simulink model "Speed_Controller_Test_forTD"  (Simulink 6.6)
settings: Solver=ode4  SolverMode=SingleTasking  StartTime=0.0  StopTime=252  FixedStep=0.01  RelTol=1e-3
InitFcn:
  | tempomat_para
StopFcn:
  | clear;
values from neighbouring files (symbols this model uses):
  A = 1.9    [tempomat_para.m]
  a_Fzg_max = 2    [tempomat_para.m]
  a_Fzg_min = -2    [tempomat_para.m]
  cw = 0.32    [tempomat_para.m]
  gang = [1 2 3 4]    [tempomat_para.m]
  gang_vec = [1 2 3 4]    [tempomat_para.m]
  i_anteil = 5    [tempomat_para.m]
  i_d = 3.42    [tempomat_para.m]
  i_g = [3.91 2.17 1.37 1.00]    [tempomat_para.m]
  lambda_gang = [1.3 1.25  1.17  1.05]    [tempomat_para.m]
  m_Fzg = 1400    [tempomat_para.m]
  M_mot_max = [130 149 163 170 168 166 162 158 150 139 123 80]    [tempomat_para.m]
  M_mot_min = [0 -40]    [tempomat_para.m]
  n_mot0 = 1000    [tempomat_para.m]
  n_mot_max = 1000:500:6500    [tempomat_para.m]
  n_mot_min = [1000 6500]    [tempomat_para.m]
  p_anteil = 100    [tempomat_para.m]
  r_dyn = 0.28    [tempomat_para.m]
  rho = 1.202    [tempomat_para.m]
  t_sch = 0.2    [tempomat_para.m]
  TI = [block '/TI']    [PSTI_callback.m]
  v_Fzg_ms0 = 0    [tempomat_para.m]
undefined symbols (not defined in the file or in its folder): Drossel_mat, getdatatypespecs
libraries: simulink x116, fzgbib x3
(part 1 of 9)
settings Model: Creator=Abel  LastModifiedBy=Justyna
settings DataIOCC: LimitDataPoints=off  SignalLoggingName=sigsOut
settings OptimizationCC: BooleanDataType=off
settings DebuggingCC: SignalResolutionControl=TryResolveAllWithWarning  InheritedTsInSrcMsg=none  MultiTaskDSMMsg=warning  MultiTaskCondExecSysMsg=none  StrictBusMsg=None
settings RTWCC: IncludeERTFirstTime=on

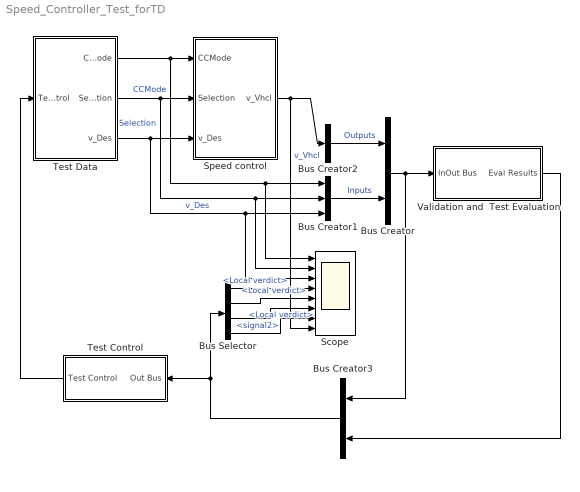
== system Speed_Controller_Test_forTD ==
  Bus Creator : BusCreator  Inputs=2
  Bus Creator1 : BusCreator  Inputs=3
  Bus Creator2 : BusCreator  Inputs=1
  Bus Creator3 : BusCreator  Orientation=left  Inputs=2
  Bus Selector : BusSelector  OutputSignals=signal2.signal1.signal1.signal1.signal1.Local verdict,signal2.signal1.signal1.signal1.signal2.Local verdict,signal2.signal1.signal2.signal1.signal1.Local verdict,signal2.signal2
  Scope : Scope  NumInputPorts=8
      settings: YMin=-5~-5~-5~-5~-5~-5~-5~-5  YMax=5~5~5~5~5~5~5~5  MaxDataPoints=5000000
  Speed control : Subsystem
  Test Control : Subsystem  Orientation=left
  Test Data : Subsystem
  Validation and  Test Evaluation : Subsystem  Description=Test evaluation system template. Create a new test evaluation system from this template.
  wires:
  Speed control/1(v_Vhcl) -> Bus Creator2/1, Scope/8  "v_Vhcl"
  Test Data/1(CCMode) -> Speed control/1(CCMode), Bus Creator1/1, Scope/1  "CCMode"
  Test Data/2(Selection) -> Speed control/2(Selection), Bus Creator1/2, Scope/2  "Selection"
  Bus Creator/1 -> Validation and  Test Evaluation/1(InOut Bus), Bus Creator3/1
  Bus Creator2/1 -> Bus Creator/1  "Outputs"
  Bus Creator1/1 -> Bus Creator/2  "Inputs"
  Test Data/3(v_Des) -> Speed control/3(v_Des), Scope/3, Bus Creator1/3  "v_Des"
  Bus Creator3/1 -> Test Control/1(Out Bus), Bus Selector/1
  Validation and  Test Evaluation/1(Eval Results) -> Bus Creator3/2
  Test Control/1(Test Control) -> Test Data/1(Test Control)
  Bus Selector/1 -> Scope/4  "<Local verdict>"
  Bus Selector/2 -> Scope/5  "<Local verdict>"
  Bus Selector/3 -> Scope/6  "<Local verdict>"
  Bus Selector/4 -> Scope/7  "<signal2>"

== system Speed_Controller_Test_forTD/Speed control ==
  CCMode : Inport
  Selection : Inport  Port=2
  v_Des : Inport  Port=3
  Bus Selector : BusSelector  OutputSignals=i_Total,n_Eng,a_Vhcl,v_Vhcl
  Compute SUC inputs : Subsystem  AncestorBlock=fzgbib/StellgroessenBerechnung BeschleunigungsBegrenzung
  Const : Constant
  Speed controller : Subsystem  AncestorBlock=fzgbib/GeschwindigkeitsRegelung
  Terminator1 : Terminator
  Terminator2 : Terminator
  Vehicle model : Subsystem
      mask Type: Vehicle Model
      mask Display: image(imread('car.jpg','jpg'),[0.05,0.2,0.9,0.6])
  "km/h -> m/s2" : Gain  Gain=1/3.6  SaturateOnIntegerOverflow=on
  "m/s2 -> km/h" : Gain  Gain=3.6  SaturateOnIntegerOverflow=on
  v_Vhcl : Outport
  wires:
  Speed controller/1(T) -> Compute SUC inputs/4(T)
  Vehicle model/1(FzgDaten) -> Bus Selector/1
  Bus Selector/1 -> Compute SUC inputs/1(i_Total)  "<i_Total>"
  Bus Selector/2 -> Compute SUC inputs/2(n_Eng)  "<n_Eng>"
  Bus Selector/3 -> Compute SUC inputs/3(a_Vhcl)  "<a_Vhcl>"
  Bus Selector/4 -> Speed controller/1(v_Vhcl), "m/s2 -> km/h"/1  "<v_Vhcl>"
  Vehicle model/2(M_Br_b) -> Terminator1/1
  Vehicle model/3(M_Mot_b) -> Terminator2/1
  Compute SUC inputs/1(SUC inputs) -> Vehicle model/1(StellgroessenTempomat), Vehicle model/3(StellgroessenFahrer)
  v_Des/1 -> "km/h -> m/s2"/1
  "m/s2 -> km/h"/1 -> v_Vhcl/1
  "km/h -> m/s2"/1 -> Speed controller/2(v_Des)
  Const/1 -> Vehicle model/2(TempomatFlag)
  Selection/1 -> Speed controller/3(Selection)
  CCMode/1 -> Speed controller/4(CCMode)

== system Speed_Controller_Test_forTD/Test Control ==
  Out Bus : Inport
  Bus Selector : BusSelector  OutputSignals=signal2.signal1.signal1.signal1.signal1.Local verdict
  Counter : Subsystem
  Memory : Memory
  OR : Logic  Operator=OR  Inputs=3  AllPortsSameDT=off  OutDataTypeMode=Boolean
  Switch : Switch  Criteria=u2 > Threshold
  error : simulink/Logic and Bit Operations/Compare To Constant  SystemSampleTime=-1  relop===  const=-1  LogicOutDataTypeMode=uint8  ZeroCross=off
  fail : simulink/Logic and Bit Operations/Compare To Constant  SystemSampleTime=-1  relop===  const=0  LogicOutDataTypeMode=uint8  ZeroCross=off
  pass : simulink/Logic and Bit Operations/Compare To Constant  SystemSampleTime=-1  relop===  const=1  LogicOutDataTypeMode=uint8  ZeroCross=off
  test case 1 : Constant
  test case 2 : Constant  Value=2
  Test Control : Outport
  wires:
  OR/1 -> Counter/1(In1), Counter/Trigger
  test case 1/1 -> Switch/3
  Out Bus/1 -> Bus Selector/1
  Switch/1 -> Test Control/1
  test case 2/1 -> Switch/1
  Counter/1(Out1) -> Switch/2
  Bus Selector/1 -> Memory/1  "<Local verdict>"
  pass/1 -> OR/1
  fail/1 -> OR/2
  error/1 -> OR/3
  Memory/1 -> pass/1, error/1, fail/1

== system Speed_Controller_Test_forTD/Test Data ==
  Test Control : Inport
  Bus Creator : BusCreator  Inputs=6
  Bus Selector : BusSelector  OutputSignals=v_Des (signal 1),v_Des (signal 4)
  Bus Selector1 : BusSelector  OutputSignals=CCMode (signal 2),CCMode (signal 5)
  Bus Selector2 : BusSelector  OutputSignals=Selection (signal 3),Selection (signal 6)
  PrecAct CCMode : MultiPortSwitch  Inputs=3  zeroidx=on
  PrecAct Selection : MultiPortSwitch  Inputs=3  zeroidx=on
  PrecAct v_Des : MultiPortSwitch  Inputs=3  zeroidx=on
  R1 Speed Control step response : Subsystem
  R2 Speed Control velocity restoration time after simple  acceleration/deceleration : Subsystem
  zero signal : Constant  Value=0
  CCMode : Outport
  Selection : Outport  Port=2
  v_Des : Outport  Port=3
  wires:
  PrecAct v_Des/1 -> v_Des/1
  zero signal/1 -> PrecAct v_Des/2, PrecAct Selection/2, PrecAct CCMode/2
  PrecAct CCMode/1 -> CCMode/1
  PrecAct Selection/1 -> Selection/1
  Bus Creator/1 -> Bus Selector/1, Bus Selector1/1, Bus Selector2/1
  Bus Selector/1 -> PrecAct v_Des/3  "<v_Des (signal 1)>"
  R1 Speed Control step response/1(v_Des) -> Bus Creator/1
  R1 Speed Control step response/2(CCMode) -> Bus Creator/2
  R1 Speed Control step response/3(Selection) -> Bus Creator/3
  R2 Speed Control velocity restoration time after simple  acceleration/deceleration/1(v_Des) -> Bus Creator/4
  R2 Speed Control velocity restoration time after simple  acceleration/deceleration/2(CCMode) -> Bus Creator/5
  R2 Speed Control velocity restoration time after simple  acceleration/deceleration/3(Selection) -> Bus Creator/6
  Bus Selector/2 -> PrecAct v_Des/4  "<v_Des (signal 4)>"
  Bus Selector1/1 -> PrecAct CCMode/3  "<CCMode (signal 2)>"
  Bus Selector1/2 -> PrecAct CCMode/4  "<CCMode (signal 5)>"
  Bus Selector2/1 -> PrecAct Selection/3  "<Selection (signal 3)>"
  Bus Selector2/2 -> PrecAct Selection/4  "<Selection (signal 6)>"
  Test Control/1 -> PrecAct v_Des/1, PrecAct CCMode/1, PrecAct Selection/1

== system Speed_Controller_Test_forTD/Validation and  Test Evaluation ==
  InOut Bus : Inport
  Arbitration : Subsystem
  Bus Creator1 : BusCreator  Inputs=2
  Bus Creator2 : BusCreator  Inputs=2
  Bus Selector1 : BusSelector  OutputSignals=signal1.signal1.signal1.Local verdict,signal1.signal1.signal2.Local verdict,signal2.signal1.signal1.Local verdict
  R1 Speed Control step response : Subsystem  Description=Requirement template. Create a new requirement from this template.
  R2 Speed Control velocity restoration time after simple  acceleration/deceleration : Subsystem  Description=Requirement template. Create a new requirement from this template.
  Signal Conversion : SignalConversion  ConversionOutput=Bus copy
  Eval Results : Outport
  wires:
  Signal Conversion/1 -> R1 Speed Control step response/1(InOut Bus), R2 Speed Control velocity restoration time after simple  acceleration/deceleration/1(InOut Bus)
  R1 Speed Control step response/1(Test Info) -> Bus Creator2/1
  InOut Bus/1 -> Signal Conversion/1
  Bus Creator2/1 -> Bus Selector1/1, Bus Creator1/1
  R2 Speed Control velocity restoration time after simple  acceleration/deceleration/1(Test Info) -> Bus Creator2/2
  Bus Selector1/1 -> Arbitration/1(In1)  "<Local verdict>"
  Bus Selector1/2 -> Arbitration/2(In2)  "<Local verdict>"
  Bus Selector1/3 -> Arbitration/3(In3)  "<Local verdict>"
  Bus Creator1/1 -> Eval Results/1
  Arbitration/1(Out1) -> Bus Creator1/2

== system Speed_Controller_Test_forTD/Speed control/Compute SUC inputs ==
  note: M_Abtr_w_Temp [Nm]
      | (Abtriebswunschmoment _Tempomat)
  note: n_Mot [1/min]
      | (Motordrehzahl)
  note: a_Fzg [m/ss]
      | (Fzg.beschleunigung)
  i_Total : Inport
  n_Eng : Inport  Port=2
  a_Vhcl : Inport  Port=3
  T : Inport  Port=4
  Constant1 : Constant  Value=0
  Gain : Gain  Gain=-1  SaturateOnIntegerOverflow=on
  Logical Operator : Logic  Operator=NOT  Inputs=1
  Mux : Mux  Inputs=2
  Oneway-Filter : Subsystem  mask(Oneway Filter){zk=2}
      mask prompts: zk "Filterkonstante"
      mask help: Filtert Signal mit Zeitkonstante zk nur, wenn kein Sprung auf Null von oben.
      mask Display: plot(0,0,100,100,[0 10 20 30 40 50 60 60 100],[0 0 30 50 60 65 67 0 0])
  Product : Product  Inputs=*/  SaturateOnIntegerOverflow=on  InputSameDT=on
  Relational Operator : RelationalOperator  InputSameDT=on
  Saturation : Saturate  UpperLimit=m_Fzg*a_Fzg_max*r_dyn  LowerLimit=m_Fzg*a_Fzg_min*r_dyn
  Schleppmoment : Lookup  InputValues=n_mot_min  OutputValues=M_mot_min  SaturateOnIntegerOverflow=on
  Sum : Sum  SaturateOnIntegerOverflow=on  InputSameDT=on
  Switch : Switch  Threshold=0.5  SaturateOnIntegerOverflow=on  InputSameDT=on
  Switch1 : Switch  Threshold=0.5  SaturateOnIntegerOverflow=on  InputSameDT=on
  neg_Beschleunigungsbegrenzung : Subsystem
  pos_Beschleunigungsbegrenzung : Subsystem
  SUC inputs : Outport  InitialOutput=0
  wires:
  Schleppmoment/1 -> Relational Operator/2, Sum/1, Switch/3
  Relational Operator/1 -> Logical Operator/1, Switch/2
  Constant1/1 -> Switch1/3
  Logical Operator/1 -> Switch1/2
  Mux/1 -> SUC inputs/1
  neg_Beschleunigungsbegrenzung/1(M_Br3) -> Oneway-Filter/1(in)
  i_Total/1 -> Product/2
  Gain/1 -> Sum/2
  Sum/1 -> Switch1/1
  Switch/1 -> pos_Beschleunigungsbegrenzung/1(M_Mot_v)
  pos_Beschleunigungsbegrenzung/1(M_Mot3) -> Mux/1  "T_Engine"
  a_Vhcl/1 -> neg_Beschleunigungsbegrenzung/2(a_Fzg_mss), pos_Beschleunigungsbegrenzung/2(a_Fzg_mss)
  n_Eng/1 -> Schleppmoment/1, pos_Beschleunigungsbegrenzung/3("n_Mot ")
  Product/1 -> Relational Operator/1, Switch/1
  Switch1/1 -> neg_Beschleunigungsbegrenzung/1(M_Br_v)
  T/1 -> Saturation/1
  Saturation/1 -> Product/1, Gain/1
  Oneway-Filter/1("out ") -> neg_Beschleunigungsbegrenzung/3(M_Br_n), Mux/2  "T_Brake"

== system Speed_Controller_Test_forTD/Speed control/Speed controller ==
  note: v_soll [m/s] (Sollgeschw.)
  note: v_Fzg [m/s] (Istgeschw.)
  note: M_Abtr_w_GR [Nm]
      | (Abtriebswunschmoment _GR)
  v_Vhcl : Inport
  v_Des : Inport  Port=2
  Selection : Inport  Port=3
  CCMode : Inport  Port=4
  Constant : Constant  Value=0
  Fcn2 : Fcn  Expr=u==2
  Fcn3 : Fcn  Expr=u!=ueberdrueckt
  Logical Operator : Logic
  Regler : Subsystem
  Stoergroessenkompensation : Subsystem
  Sum : Sum  Inputs=+-  SaturateOnIntegerOverflow=on  InputSameDT=on
  Sum2 : Sum  Inputs=2  SaturateOnIntegerOverflow=on  InputSameDT=on
  Switch : Switch  Threshold=0.5  SaturateOnIntegerOverflow=on  InputSameDT=on
  Switch1 : Switch  Threshold=0.5  SaturateOnIntegerOverflow=on  InputSameDT=on
  T : Outport  InitialOutput=0
  wires:
  Logical Operator/1 -> Stoergroessenkompensation/3(GR_aktiv_l)
  Regler/1("u_R ") -> Sum2/2
  Stoergroessenkompensation/1(u_s) -> Sum2/1
  v_Vhcl/1 -> Stoergroessenkompensation/1(v_Fzg), Switch1/1
  Sum/1 -> Regler/1(d_v)
  Constant/1 -> Switch/3
  Switch1/1 -> Sum/2
  Fcn2/1 -> Logical Operator/1
  Selection/1 -> Fcn2/1
  CCMode/1 -> Fcn3/1
  Fcn3/1 -> Logical Operator/2, Switch1/2, Switch/2
  Switch/1 -> T/1
  Sum2/1 -> Switch/1
  v_Des/1 -> Switch1/3, Sum/1, Stoergroessenkompensation/2(v_soll)

== system Speed_Controller_Test_forTD/Speed control/Vehicle model ==
  note: i_Gesamt
      | n_mot
      | a_Fzg_mss
      | v_Fzg_ms
      | Gang_i
  StellgroessenTempomat : Inport  Orientation=left
  TempomatFlag : Inport  Orientation=left  Port=2
  StellgroessenFahrer : Inport  Orientation=left  Port=3
  Bremsmomenten beschaenkung : fzgbib/Bremsmomenten beschraenkung  Orientation=left  SystemSampleTime=-1
  Bus Creator : BusCreator  Orientation=left  Inputs=5
  Fahrzeugmodell : Subsystem  Orientation=left  AncestorBlock=fzgbib/Fahrzeugmodell
  Gangberechnung : fzgbib/Gangberechnung  Orientation=left  SystemSampleTime=-1
  M_Mot M_Br : Demux  Orientation=left  Outputs=2
  Motormoment beschraenkung : fzgbib/Motormoment beschraenkung  Orientation=left  SystemSampleTime=-1
  SG-Koordinator : Subsystem  Orientation=left
  Terminator : Terminator
  FzgDaten : Outport  Orientation=left
  M_Br_b : Outport  Orientation=left  Port=2
  M_Mot_b : Outport  Orientation=left  Port=3
  wires:
  M_Mot M_Br/1 -> Gangberechnung/1, Motormoment beschraenkung/1
  Fahrzeugmodell/5(a_Fzg_mss) -> Bus Creator/3  "a_Vhcl"
  Fahrzeugmodell/1(v_Fzg_ms) -> Bus Creator/4  "v_Vhcl"
  Motormoment beschraenkung/1 -> Fahrzeugmodell/2(M_Mot_b), M_Mot_b/1
  M_Mot M_Br/2 -> Bremsmomenten beschaenkung/1
  Fahrzeugmodell/4(Gang_i) -> Gangberechnung/3, Bus Creator/5  "Gang_i"
  Fahrzeugmodell/6("DK_Stellung ") -> Terminator/1
  Fahrzeugmodell/3(n_Mot) -> Gangberechnung/2, Motormoment beschraenkung/2, Bus Creator/2  "n_Eng"
  Fahrzeugmodell/2(i_gesamt) -> Bus Creator/1  "i_Total"
  Gangberechnung/1 -> Fahrzeugmodell/3(Gang_w)
  SG-Koordinator/1(Momente) -> M_Mot M_Br/1
  Bremsmomenten beschaenkung/1 -> Fahrzeugmodell/1(M_Br_b), M_Br_b/1
  StellgroessenTempomat/1 -> SG-Koordinator/1(Tempomat)
  TempomatFlag/1 -> SG-Koordinator/2(TempomatFlag)
  StellgroessenFahrer/1 -> SG-Koordinator/3(Fahrer)
  Bus Creator/1 -> FzgDaten/1

== system Speed_Controller_Test_forTD/Test Control/Counter ==
  In1 : Inport
  Trigger : TriggerPort
  " 1" : DataTypeConversion  Orientation=down
  Add : Sum  OutScaling=2^-10
  Memory : Memory  Orientation=left  InheritSampleTime=on
  Number of triggers : Constant  Value=2
  Relational Operator1 : RelationalOperator  Operator===  LogicOutDataTypeMode=Boolean
  Scope1 : Scope  NumInputPorts=4
      settings: YMin=182.932~-5~-5~-5  YMax=202.188~5~5~5  SaveName=ScopeData14  MaxDataPoints=5000000
  Out1 : Outport
  wires:
  In1/1 -> Add/1, Scope1/2
  Number of triggers/1 -> Relational Operator1/2
  Relational Operator1/1 -> Out1/1
  Add/1 -> " 1"/1, Relational Operator1/1, Scope1/3
  Memory/1 -> Add/2
  " 1"/1 -> Memory/1

== system Speed_Controller_Test_forTD/Test Data/R1 Speed Control step response ==
  Complete step & CC active + no target & Speed Control active : Subsystem  Description=Preconditions template. Create new preconditions blocks using this template.
  v_Des : Outport
  CCMode : Outport  Port=2
  Selection : Outport  Port=3
  wires:
  Complete step & CC active + no target & Speed Control active/1(v_Des) -> v_Des/1  "v_Des"
  Complete step & CC active + no target & Speed Control active/2(CCMode) -> CCMode/1  "CCMode"
  Complete step & CC active + no target & Speed Control active/3(Selection) -> Selection/1  "Selection"

== system Speed_Controller_Test_forTD/Test Data/R2 Speed Control velocity restoration time after simple  acceleration/deceleration ==
  " CC active + no target & Speed Control active & V_Des increases/decreases  7 times by 1 unit" : Subsystem  Description=Preconditions template. Create new preconditions blocks using this template.
  v_Des : Outport
  CCMode : Outport  Port=2
  Selection : Outport  Port=3
  wires:
  " CC active + no target & Speed Control active & V_Des increases/decreases  7 times by 1 unit"/2(CCMode) -> CCMode/1  "CCMode"
  " CC active + no target & Speed Control active & V_Des increases/decreases  7 times by 1 unit"/3(Selection) -> Selection/1  "Selection"
  " CC active + no target & Speed Control active & V_Des increases/decreases  7 times by 1 unit"/1(v_Des) -> v_Des/1  "v_Des"

== system Speed_Controller_Test_forTD/Validation and  Test Evaluation/Arbitration ==
  In1 : Inport
  In2 : Inport  Port=2
  In3 : Inport  Port=3
  Collect Verdicts : MinMax  Inputs=4
  Memory : Memory  Orientation=left  X0=2
  Out1 : Outport
  wires:
  Memory/1 -> Collect Verdicts/4
  Collect Verdicts/1 -> Out1/1, Memory/1
  In1/1 -> Collect Verdicts/1
  In2/1 -> Collect Verdicts/2
  In3/1 -> Collect Verdicts/3

== system Speed_Controller_Test_forTD/Validation and  Test Evaluation/R1 Speed Control step response ==
  InOut Bus : Inport
  Bus Creator : BusCreator  Inputs=2
  Complete step & CC active + no target & Speed Control active : Subsystem  Description=Preconditions template. Create new preconditions blocks using this template.
  Maximum overshoot < 5 &  Steady state error < 5 : Subsystem  Description=Assertions template. Create a new assertions block from this template.
  Test Info : Outport
  wires:
  InOut Bus/1 -> Complete step & CC active + no target & Speed Control active/1(InOut Bus), Maximum overshoot < 5 &  Steady state error < 5/2(InOut Bus)
  Maximum overshoot < 5 &  Steady state error < 5/1(VF info) -> Bus Creator/1
  Bus Creator/1 -> Test Info/1
  Complete step & CC active + no target & Speed Control active/1(Activate) -> Maximum overshoot < 5 &  Steady state error < 5/1(Precond), Bus Creator/2

== system Speed_Controller_Test_forTD/Validation and  Test Evaluation/R2 Speed Control velocity restoration time after simple  acceleration/deceleration ==
  InOut Bus : Inport
  Bus Creator : BusCreator  Inputs=2
  CC active + no target & Speed Control active & step of V_Des = |1|  with time periods >= 7s : Subsystem  Description=Preconditions template. Create new preconditions blocks using this template.
  after (6 seconds)  |V_Des-V_Vhcl <= 1.4| : Subsystem  Description=Assertions template. Create a new assertions block from this template.
  Test Info : Outport
  wires:
  InOut Bus/1 -> CC active + no target & Speed Control active & step of V_Des = |1|  with time periods >= 7s/1(InOut Bus), after (6 seconds)  |V_Des-V_Vhcl <= 1.4|/2(InOut Bus)
  after (6 seconds)  |V_Des-V_Vhcl <= 1.4|/1(VF info) -> Bus Creator/1
  Bus Creator/1 -> Test Info/1
  CC active + no target & Speed Control active & step of V_Des = |1|  with time periods >= 7s/1(Activate) -> after (6 seconds)  |V_Des-V_Vhcl <= 1.4|/1(Precond), Bus Creator/2

== system Speed_Controller_Test_forTD/Speed control/Compute SUC inputs/Oneway-Filter ==
  note: 21.5.1997/Hoetzer/FKFS
  in : Inport
  1/T : Fcn  Expr=1/u
  Fcn : Fcn  Expr=u[1]<-0.01
  Fcn1 : Fcn  Expr=u[1]<0.01
  Grenze3 : Constant  Value=zk
  Grenze4 : Constant  Value=0.1
  Integrator : Integrator
  Logical Operator : Logic  Operator=OR
  Logical Operator1 : Logic
  Product : Product  SaturateOnIntegerOverflow=on  InputSameDT=on
  Reglerabweichung : Sum  Inputs=-+  SaturateOnIntegerOverflow=on  InputSameDT=on
  Relational Operator1 : RelationalOperator  InputSameDT=on
  Switch : Switch  Threshold=0.5  SaturateOnIntegerOverflow=on  InputSameDT=on
  reale Ableitung : TransferFcn  Numerator=[1 0]  Denominator=[0.1 1]
  "out " : Outport  InitialOutput=0
  wires:
  Relational Operator1/1 -> Logical Operator1/2
  Fcn/1 -> Logical Operator1/1
  reale Ableitung/1 -> Fcn/1
  Grenze3/1 -> Switch/3
  Grenze4/1 -> Switch/1
  in/1 -> Relational Operator1/2, Fcn1/1, reale Ableitung/1, Reglerabweichung/2
  1/T/1 -> Product/2
  Reglerabweichung/1 -> Product/1
  Switch/1 -> 1/T/1
  Logical Operator/1 -> Switch/2
  Product/1 -> Integrator/1
  Integrator/1 -> Relational Operator1/1, Reglerabweichung/1, "out "/1
  Fcn1/1 -> Logical Operator/2
  Logical Operator1/1 -> Logical Operator/1

== system Speed_Controller_Test_forTD/Speed control/Compute SUC inputs/neg_Beschleunigungsbegrenzung ==
  note: Das Bremsmoment wird solange durchgereicht, solange die Beschleunigung > -2 ist.
      | Im anderen Fall wird das in diesem Fall gespeicherte Bremsmoment durchgereicht.
  M_Br_v : Inport
  a_Fzg_mss : Inport  Port=2
  M_Br_n : Inport  Port=3
  Constant1 : Constant  Value=a_Fzg_min
  Data Store Memory : DataStoreMemory  DataStoreName=M_Br2  InitialValue=0
  Data Store Read : DataStoreRead  DataStoreName=M_Br2  SampleTime=-1
  Gangspeicher : Memory  X0=1
  Logical Operator : Logic  Operator=OR
  Logical Operator1 : Logic  Orientation=down  Operator=NOT  Inputs=1
  Relational Operator : RelationalOperator  Operator=>  InputSameDT=on
  Relational Operator1 : RelationalOperator  Operator=<=  InputSameDT=on
  Reset M_Br2 : Subsystem  TreatAsAtomicUnit=on
  Switch : Switch  Threshold=0.5  SaturateOnIntegerOverflow=on  InputSameDT=on
  tw5 : ToWorkspace  VariableName=b_l  SaveFormat=Array
      settings: MaxDataPoints=speicher
  tw6 : ToWorkspace  VariableName=M_Br2  SaveFormat=Array
      settings: MaxDataPoints=speicher
  tw7 : ToWorkspace  VariableName=M_Br1  SaveFormat=Array
      settings: MaxDataPoints=speicher
  M_Br3 : Outport  InitialOutput=0
  wires:
  Switch/1 -> M_Br3/1
  Constant1/1 -> Relational Operator/2
  Relational Operator1/1 -> Logical Operator/2
  Data Store Read/1 -> Switch/3, tw6/1, Relational Operator1/2
  Logical Operator/1 -> Gangspeicher/1
  Gangspeicher/1 -> Switch/2, tw5/1
  M_Br_n/1 -> Reset M_Br2/1(M_Br_n)
  M_Br_v/1 -> Switch/1, tw7/1, Relational Operator1/1
  Relational Operator/1 -> Logical Operator/1, Logical Operator1/1
  Logical Operator1/1 -> Reset M_Br2/Enable
  a_Fzg_mss/1 -> Relational Operator/1, Reset M_Br2/2(a_Fzg_mss)

== system Speed_Controller_Test_forTD/Speed control/Compute SUC inputs/pos_Beschleunigungsbegrenzung ==
  note: Das Bremsmoment wird solange durchgereicht, solange die Beschleunigung > -2 ist.
      | Im anderen Fall wird das in diesem Fall gespeicherte Bremsmoment durchgereicht.
  M_Mot_v : Inport
  a_Fzg_mss : Inport  Port=2
  "n_Mot " : Inport  Port=3
  Constant1 : Constant  Value=a_Fzg_max
  Data Store Memory : DataStoreMemory  DataStoreName=M_Mot2  InitialValue=0
  Data Store Read : DataStoreRead  DataStoreName=M_Mot2  SampleTime=-1
  Gangspeicher : Memory  X0=1
  Logical Operator : Logic  Operator=OR
  Logical Operator1 : Logic  Orientation=down  Operator=NOT  Inputs=1
  MinMax : MinMax  Inputs=2  SaturateOnIntegerOverflow=on  InputSameDT=on
  Relational Operator : RelationalOperator  Operator=<  InputSameDT=on
  Relational Operator1 : RelationalOperator  Operator=<=  InputSameDT=on
  Reset M_Mot2 : Subsystem  TreatAsAtomicUnit=on
  Switch : Switch  Threshold=0.5  SaturateOnIntegerOverflow=on  InputSameDT=on
  maximales Motormoment : Lookup  InputValues=[0 n_mot_max]  OutputValues=[M_mot_max(1) M_mot_max]  SaturateOnIntegerOverflow=on
  tw5 : ToWorkspace  VariableName=b_l2  SaveFormat=Array
      settings: MaxDataPoints=speicher
  tw6 : ToWorkspace  VariableName=M_Mot2  SaveFormat=Array
      settings: MaxDataPoints=speicher
  tw7 : ToWorkspace  VariableName=M_Mot1  SaveFormat=Array
      settings: MaxDataPoints=speicher
  M_Mot3 : Outport  InitialOutput=0
  wires:
  Switch/1 -> M_Mot3/1
  Constant1/1 -> Relational Operator/2
  Relational Operator1/1 -> Logical Operator/2
  Data Store Read/1 -> Switch/3, tw6/1, Relational Operator1/2
  Logical Operator/1 -> Gangspeicher/1
  Gangspeicher/1 -> Switch/2, tw5/1
  M_Mot_v/1 -> Switch/1, tw7/1, Relational Operator1/1, MinMax/1
  Relational Operator/1 -> Logical Operator/1, Logical Operator1/1
  Logical Operator1/1 -> Reset M_Mot2/Enable
  a_Fzg_mss/1 -> Relational Operator/1
  MinMax/1 -> Reset M_Mot2/1(M_Mot_n)
  "n_Mot "/1 -> maximales Motormoment/1
  maximales Motormoment/1 -> MinMax/2

== system Speed_Controller_Test_forTD/Speed control/Speed controller/Regler ==
  d_v : Inport
  Integrator : Integrator  LimitOutput=on  UpperSaturationLimit=2000  LowerSaturationLimit=-2000
  P_Anteil : Gain  Gain=p_anteil  SaturateOnIntegerOverflow=on
  Sum : Sum  SaturateOnIntegerOverflow=on  InputSameDT=on
  "m/s -> km/h1" : Gain  Gain=i_anteil  SaturateOnIntegerOverflow=on
  "u_R " : Outport  InitialOutput=0
  wires:
  Sum/1 -> "u_R "/1
  P_Anteil/1 -> Sum/1
  "m/s -> km/h1"/1 -> Integrator/1
  d_v/1 -> P_Anteil/1, "m/s -> km/h1"/1
  Integrator/1 -> Sum/2

== system Speed_Controller_Test_forTD/Speed control/Speed controller/Stoergroessenkompensation ==
  v_Fzg : Inport
  v_soll : Inport  Port=2
  GR_aktiv_l : Inport  Port=3
  Luft- und Rollwiderstand : Subsystem
  P-Anteil : Gain  Gain=3000  SaturateOnIntegerOverflow=on
  P-Anteil1 : Gain  Gain=m_Fzg  SaturateOnIntegerOverflow=on
  Sollverhalten Fahrzeug mit P-Regler1 : Subsystem
  Sum : Sum  Inputs=2  SaturateOnIntegerOverflow=on  InputSameDT=on
  Sum1 : Sum  Inputs=2  SaturateOnIntegerOverflow=on  InputSameDT=on
  Sum2 : Sum  Inputs=+-  SaturateOnIntegerOverflow=on  InputSameDT=on
  r_dyn : Gain  Gain=r_dyn  SaturateOnIntegerOverflow=on
  reale Ableitung : TransferFcn  Numerator=[1 0]  Denominator=[0.5 1]
  u_s : Outport  InitialOutput=0
  wires:
  Sum1/1 -> Sum/2
  Luft- und Rollwiderstand/1(M_G) -> Sum/1
  P-Anteil/1 -> Sum1/2
  P-Anteil1/1 -> Sum1/1
  Sollverhalten Fahrzeug mit P-Regler1/1(v_Fzg1) -> Sum2/1
  r_dyn/1 -> P-Anteil1/1
  GR_aktiv_l/1 -> Sollverhalten Fahrzeug mit P-Regler1/3(GR_aktiv_l)
  reale Ableitung/1 -> r_dyn/1
  v_soll/1 -> Sollverhalten Fahrzeug mit P-Regler1/1(v_soll)
  Sum2/1 -> reale Ableitung/1, P-Anteil/1
  v_Fzg/1 -> Sollverhalten Fahrzeug mit P-Regler1/2(v_Fzg), Sum2/2, Luft- und Rollwiderstand/1(v_Fzg)
  Sum/1 -> u_s/1

== system Speed_Controller_Test_forTD/Speed control/Vehicle model/Fahrzeugmodell ==
  M_Br_b : Inport
  M_Mot_b : Inport  Port=2
  Gang_w : Inport  Port=3
  Drosselklappenstellung : Subsystem
  Fahrwiderstaende : Subsystem
  Fahrzeugdynamik : Subsystem
  tw6 : ToWorkspace  VariableName=v_Fzg_kmh  SaveFormat=Array
      settings: MaxDataPoints=speicher
  v_Fzg_ms : Outport  InitialOutput=0
  i_gesamt : Outport  Port=2  InitialOutput=0
  n_Mot : Outport  Port=3  InitialOutput=0
  Gang_i : Outport  Port=4  InitialOutput=0
  a_Fzg_mss : Outport  Port=5  InitialOutput=0
  "DK_Stellung " : Outport  Port=6  InitialOutput=0
  wires:
  Fahrwiderstaende/7(schalt_l) -> Drosselklappenstellung/3(schalt_l)
  Fahrzeugdynamik/4(a_Fzg_mss) -> a_Fzg_mss/1
  Fahrzeugdynamik/1(v_Fzg_kmh) -> tw6/1
  Fahrwiderstaende/6(Gang_i) -> Gang_i/1, Fahrzeugdynamik/6(Gang_i)
  Fahrzeugdynamik/3(n_Mot) -> Drosselklappenstellung/1(n_mot), n_Mot/1
  Fahrzeugdynamik/2(v_Fzg_ms) -> Fahrwiderstaende/4(v_Fzg_ms), v_Fzg_ms/1
  Drosselklappenstellung/1(DK_Stellung [Grad]) -> "DK_Stellung "/1
  Fahrwiderstaende/1(F_A) -> Fahrzeugdynamik/1(F_A)
  Fahrwiderstaende/4(F_Brems) -> Fahrzeugdynamik/4(F_Brems)
  Fahrwiderstaende/2(F_L) -> Fahrzeugdynamik/2(F_L)
  Fahrwiderstaende/3(F_R) -> Fahrzeugdynamik/3(F_R)
  M_Mot_b/1 -> Drosselklappenstellung/2(M_Mot_b), Fahrwiderstaende/1(M_Mot_b)
  Gang_w/1 -> Fahrwiderstaende/3(Gang_w)
  M_Br_b/1 -> Fahrwiderstaende/2(M_Br_b)
  Fahrwiderstaende/5(i_gesamt) -> Fahrzeugdynamik/5(i_gesamt), i_gesamt/1

== system Speed_Controller_Test_forTD/Speed control/Vehicle model/SG-Koordinator ==
  note: TempomatFlag = 1 => Tempomat hat Priorität
  note: TempomatFlag = 0 => Fahrer hat Priorität
  Tempomat : Inport
  TempomatFlag : Inport  Port=2
  Fahrer : Inport  Port=3
  Bus Selector : BusSelector  OutputSignals=T_Engine,T_Brake
  Bus Selector1 : BusSelector  OutputSignals=T_Engine,T_Brake
  Constant3 : Constant
  Multiport Switch : MultiPortSwitch  Inputs=2  SaturateOnIntegerOverflow=on  InputSameDT=on
  Mux : Mux  Inputs=2
  Mux1 : Mux  Inputs=2
  Sum : Sum  SaturateOnIntegerOverflow=on  InputSameDT=on
  Momente : Outport  InitialOutput=0
  wires:
  Multiport Switch/1 -> Momente/1
  Sum/1 -> Multiport Switch/1
  Constant3/1 -> Sum/2
  TempomatFlag/1 -> Sum/1
  Bus Selector/1 -> Mux/1  "<T_Engine>"
  Bus Selector/2 -> Mux/2  "<T_Brake>"
  Tempomat/1 -> Bus Selector/1
  Mux/1 -> Multiport Switch/3
  Bus Selector1/1 -> Mux1/1  "<T_Engine>"
  Bus Selector1/2 -> Mux1/2  "<T_Brake>"
  Fahrer/1 -> Bus Selector1/1
  Mux1/1 -> Multiport Switch/2

== system Speed_Controller_Test_forTD/Test Data/R1 Speed Control step response/Complete step & CC active + no target & Speed Control active ==
  Active : Constant  Value=2
  Active + no target : Constant  Value=2
  Generate Step : Step  Time=60  Before=80  After=100  SampleTime=0
  Scope2 : Scope  NumInputPorts=3
      settings: YMin=40~-5~-5  YMax=100~5~5  MaxDataPoints=11115000
  v_Des : Outport
  CCMode : Outport  Port=2
  Selection : Outport  Port=3
  wires:
  Active + no target/1 -> CCMode/1
  Active/1 -> Selection/1
  Generate Step/1 -> Scope2/1, v_Des/1

== system Speed_Controller_Test_forTD/Test Data/R2 Speed Control velocity restoration time after simple  acceleration/deceleration/ CC active + no target & Speed Control active & V_Des increases/decreases  7 times by 1 unit ==
  Active : Constant  Value=2
  Active + no target : Constant  Value=2
  V_Des increases/decreases  7 times by 1 unit : Subsystem  Description=Preconditions template. Create new preconditions blocks using this template.
  v_Des : Outport
  CCMode : Outport  Port=2
  Selection : Outport  Port=3
  wires:
  Active + no target/1 -> CCMode/1
  Active/1 -> Selection/1
  V_Des increases/decreases  7 times by 1 unit/1(v_Des) -> v_Des/1

== system Speed_Controller_Test_forTD/Validation and  Test Evaluation/R1 Speed Control step response/Complete step & CC active + no target & Speed Control active ==
  InOut Bus : Inport
  Active : Constant  Value=2
  Active + no target : Constant  Value=2
  Bus Selector : BusSelector  OutputSignals=Inputs.v_Des,Outputs.v_Vhcl,Inputs.CCMode,Inputs.Selection
  CC active & no target : Subsystem  mask(Range - Gap Absolute Tolerance){GorR=Range, AbsoluteTolerance=0}
      mask prompts: GorR "Use range or gap"; AbsoluteTolerance "Absolute Tolerance"
      mask help: Check that a signal stays inside a range or outside a gap around a reference signal. Specify the range or the gap absolute to the reference signal.
      mask init:
      | if max(get_param(gcb,'GorR') == ' ') % Gap
      |     helpVariable1 = '~=';
      | else % Range
      |     helpVariable1 = '==';
      | end
      | set_param([gcb '/Relational Operator'],'Operator',helpVariable1);
      mask StyleString: popup(Range|Gap  ),edit
      mask Display:
      | port_label('output',1,'A');
      | port_label('input',1,'Sig');
      | port_label('input',2,'Ref');
      | text(0.40,0.53,'+');
      | text(0.415,0.46,'-');
      | text(0.5,0.5,num2str(AbsoluteTolerance));
      | text(0.05,0.5,helpVariable1);
  Complete step : Constant
  Complete step detection : Subsystem  mask(Complete step detection){Param=0}
      mask prompts: Param "Mask Parameter 1:"
  PS : Subsystem  mask(Feature layer: preconditions synchronization){NoTI=2, NoTDD=0, NoTID=1, TIdel=[0  0], TDDdel=[]}
      mask prompts: NoTI "Time-independent features identifiable with or without a delay (TI)"; NoTDD "Triggered features identifiable with determinate delay or without a delay (TDD)"; NoTID "Triggered features identifiable with indeterminate delay (TID)"; TIdel "Time-independent features delays (in time steps). E.g. [0 1 0] for 3 features"; TDDdel "Triggered features delays (in time steps). E.g. [0 0] for 2 features"
      mask help: Use this block for synchronizing the precondition features. For changing the block inputs, use the parameters below. The output must be used for assertions activation.
      mask init:
      | PS_init(gcb);
      mask StyleString: popup(0|1|2|3|4|5|6|7|8|9),popup(0|1|2|3|4|5|6|7|8|9),popup(0|1|2|3|4|5|6|7|8|9),edit,edit
      mask CallbackString:
      | PSTI_callback(gcb);|PSTDD_callback(gcb);|PSTID_callback(gcb);|NoTI = str2double(get_param(gcb,'NoTI'));
      | TIdel = str2num(get_param(gcb,'TIdel'));
      | if NoTI ~= length(TIdel) && NoTI ~= 0
      |     error(['The number of delays entered (' num2str(length(TIdel)) ') does not correspond to the above specified number of time-independent features (' num2str(NoTI) ').']);
      | end|NoTDD = str2double(get_param(gcb,'NoTDD'));
      | TDDdel = str2num(get_param(gcb,'TDDdel'));
      | if NoTDD ~= length(TDDdel) && NoTDD ~= 0
      |     error(['The number of delays entered (' num2str(length(TDDdel)) ') does not correspond to the above specified number of triggered features with constant delay (' num2str(NoTDD) ').']);
      | end
  Range - Gap Absolute tolerance Precond : Subsystem  mask(Range - Gap Absolute Tolerance){GorR=Range, AbsoluteTolerance=0}
      mask prompts: GorR "Use range or gap"; AbsoluteTolerance "Absolute Tolerance"
      mask help: Check that a signal stays inside a range or outside a gap around a reference signal. Specify the range or the gap absolute to the reference signal.
      mask init:
      | if max(get_param(gcb,'GorR') == ' ') % Gap
      |     helpVariable1 = '~=';
      | else % Range
      |     helpVariable1 = '==';
      | end
      | set_param([gcb '/Relational Operator'],'Operator',helpVariable1);
      mask StyleString: popup(Range|Gap  ),edit
      mask Display:
      | port_label('output',1,'A');
      | port_label('input',1,'Sig');
      | port_label('input',2,'Ref');
      | text(0.40,0.53,'+');
      | text(0.415,0.46,'-');
      | text(0.5,0.5,num2str(AbsoluteTolerance));
      | text(0.05,0.5,helpVariable1);
  Speed control active : Subsystem  mask(Range - Gap Absolute Tolerance){GorR=Range, AbsoluteTolerance=0}
      mask prompts: GorR "Use range or gap"; AbsoluteTolerance "Absolute Tolerance"
      mask help: Check that a signal stays inside a range or outside a gap around a reference signal. Specify the range or the gap absolute to the reference signal.
      mask init:
      | if max(get_param(gcb,'GorR') == ' ') % Gap
      |     helpVariable1 = '~=';
      | else % Range
      |     helpVariable1 = '==';
      | end
      | set_param([gcb '/Relational Operator'],'Operator',helpVariable1);
      mask StyleString: popup(Range|Gap  ),edit
      mask Display:
      | port_label('output',1,'A');
      | port_label('input',1,'Sig');
      | port_label('input',2,'Ref');
      | text(0.40,0.53,'+');
      | text(0.415,0.46,'-');
      | text(0.5,0.5,num2str(AbsoluteTolerance));
      | text(0.05,0.5,helpVariable1);
  Activate : Outport
  wires:
  Complete step detection/1(R) -> PS/1(R TID1)
  Complete step detection/2(T) -> PS/2(T TID1)
  Complete step detection/3(Complete step) -> Range - Gap Absolute tolerance Precond/1(Signal)
  Complete step/1 -> Range - Gap Absolute tolerance Precond/2(Reference)
  Range - Gap Absolute tolerance Precond/1(Activate) -> PS/3(A TID1)
  PS/1(Precond) -> Activate/1
  InOut Bus/1 -> Bus Selector/1
  Bus Selector/1 -> Complete step detection/1(Step)  "<v_Des>"
  Bus Selector/2 -> Complete step detection/2(Step response)  "<v_Vhcl>"
  Bus Selector/3 -> CC active & no target/1(Signal)  "<CCMode>"
  Active + no target/1 -> CC active & no target/2(Reference)
  CC active & no target/1(Activate) -> PS/4(A TI1)
  Active/1 -> Speed control active/2(Reference)
  Speed control active/1(Activate) -> PS/5(A TI2)
  Bus Selector/4 -> Speed control active/1(Signal)  "<Selection>"

== system Speed_Controller_Test_forTD/Validation and  Test Evaluation/R1 Speed Control step response/Maximum overshoot < 5 &  Steady state error < 5 ==
  Precond : Inport
  InOut Bus : Inport  Port=2
  Abs : Abs
  Bus Creator : BusCreator  Inputs=2
  Bus Selector : BusSelector  OutputSignals=Inputs.v_Des,Outputs.v_Vhcl
  Maximum Overshoot : Constant  Value=5
  Maximum overshoot < 5 : Subsystem  mask(Bound){cm=<, Lower=1, Upper=0, Ass=[1 2], Pre=[1 2], Req=[1 2]}
      mask prompts: cm "Comparison method:"; Upper "Mask Parameter 3:"; Req "Mask Parameter 6:"
      mask help:
      | Compare a signal with a reference using the specified comparison method.
      |
      | Output verdict V and lower (LL) and upper (UL) limits for reporting.
      |
      | For '==' or '~=' use "Range - Gap"
      mask init:
      | set_param([get_param(gcb,'Parent') '/' get_param(gcb,'Name') '/Relational Operator'],'Operator',get_param(gcb,'cm'));
      | set_param(gcb,'Upper',num2str(uint8(max(get_param([get_param(gcb,'Parent') '/' get_param(gcb,'Name') '/Relational Operator'],'Operator') == '>'))));
      | set_param(gcb,'Lower',num2str(uint8(max(get_param([get_param(gcb,'Parent') '/' get_param(gcb,'Name') '/Relational Operator'],'Operator') == '<'))));
      | set_param(gcb, ...
      |           'Ass', ...
      |           ['[1 2]']);
      | set_param(gcb, ...
      |           'Pre', ...
      |           ['[1 2]']); 
      | set_param(gcb, ...
      |           'Req', ...
      |           ['[1 2]']);
      mask StyleString: popup(>|>=|<=|<),edit,edit,edit,edit,edit
      mask Display:
      | port_label('output', 1, ['V']);
      | port_label('input', 1, 'Sig');
      | port_label('input', 2, 'Ref');
      | text(0.05,0.5,get_param(get_param([get_param(gcb,'Parent') '/' get_param(gcb,'Name') '/Relational Operator'],'handle'),'Operator'));
  PAS : Subsystem  mask{AFT=TID, AFD=2}
      mask prompts: AFT "Assertion feature type:"; AFD "Assertion feature delay (in time steps)"
      mask init:
      | PAS_init(gcb);
      mask StyleString: popup(TI|TDD|TID),edit
      mask CallbackString: PAS_callback(gcb);|
  PAS1 : Subsystem  mask{AFT=TID, AFD=2}
      mask prompts: AFT "Assertion feature type:"; AFD "Assertion feature delay (in time steps)"
      mask init:
      | PAS_init(gcb);
      mask StyleString: popup(TI|TDD|TID),edit
      mask CallbackString: PAS_callback(gcb);|
  Steady state error < 5 : Subsystem  mask(Bound){cm=<, Lower=1, Upper=0, Ass=[1 2], Pre=[1 2], Req=[1 2]}
      mask prompts: cm "Comparison method:"; Upper "Mask Parameter 3:"; Req "Mask Parameter 6:"
      mask help:
      | Compare a signal with a reference using the specified comparison method.
      |
      | Output verdict V and lower (LL) and upper (UL) limits for reporting.
      |
      | For '==' or '~=' use "Range - Gap"
      mask init: same as Speed_Controller_Test_forTD/Validation and  Test Evaluation/R1 Speed Control step response/Maximum overshoot < 5 &  Steady state error < 5/Maximum overshoot < 5
      mask StyleString: popup(>|>=|<=|<),edit,edit,edit,edit,edit
      mask Display:
      | port_label('output', 1, ['V']);
      | port_label('input', 1, 'Sig');
      | port_label('input', 2, 'Ref');
      | text(0.05,0.5,get_param(get_param([get_param(gcb,'Parent') '/' get_param(gcb,'Name') '/Relational Operator'],'handle'),'Operator'));
  Steady state error : Constant  Value=5
  Step response characteristics : Subsystem  mask(Step response characteristics){MT=10, MSS=10}
      mask prompts: MT "Minimal time for signals to be constant before a step"; MSS "Minimal step size for step detection"
      mask help:
      | Detect step response characteristics and extract all the features:
      | - maximum overshoot,
      | - steady state error,
      | - rise time,
      | - settling time
  Terminator{1..4} (4 alike) : Terminator
  VF info : Outport
  wires:
  Bus Selector/1 -> Step response characteristics/1(Step)  "<v_Des>"
  Step response characteristics/1(R) -> PAS1/2(R), PAS/2(R)  "Ra"
  PAS/1(VF Info) -> Bus Creator/1
  Precond/1 -> PAS1/1(Precond), PAS/1(Precond)
  InOut Bus/1 -> Bus Selector/1
  Bus Creator/1 -> VF info/1
  Bus Selector/2 -> Step response characteristics/2(Step response)  "<v_Vhcl>"
  PAS1/1(VF Info) -> Bus Creator/2
  Maximum overshoot < 5/1(V) -> PAS/4(V)
  Maximum Overshoot/1 -> Maximum overshoot < 5/2(Reference)
  Step response characteristics/7(Maximum Overshoot) -> Abs/1
  Step response characteristics/3(Overshoot T) -> PAS/3(T)  "Ta"
  Step response characteristics/5(Steady state error T) -> PAS1/3(T)  "Ta"
  Steady state error < 5/1(V) -> PAS1/4(V)
  Steady state error/1 -> Steady state error < 5/2(Reference)
  Step response characteristics/9(Steady state error) -> Steady state error < 5/1(Signal)
  Step response characteristics/8(Settling time) -> Terminator4/1
  Step response characteristics/6(Rise time) -> Terminator3/1
  Step response characteristics/4(Settling time T) -> Terminator2/1
  Step response characteristics/2(Rise time T) -> Terminator1/1
  Abs/1 -> Maximum overshoot < 5/1(Signal)

== system Speed_Controller_Test_forTD/Validation and  Test Evaluation/R2 Speed Control velocity restoration time after simple  acceleration/deceleration/CC active + no target & Speed Control active & step of V_Des = |1|  with time periods >= 7s ==
  InOut Bus : Inport
  Active : Constant  Value=2
  Active + no target : Constant  Value=2
  Bus Selector : BusSelector  OutputSignals=Inputs.v_Des,Inputs.CCMode,Inputs.Selection
  CC active & no target : Subsystem  mask(Range - Gap Absolute Tolerance){GorR=Range, AbsoluteTolerance=0}
      mask prompts: GorR "Use range or gap"; AbsoluteTolerance "Absolute Tolerance"
      mask help: Check that a signal stays inside a range or outside a gap around a reference signal. Specify the range or the gap absolute to the reference signal.
      mask init:
      | if max(get_param(gcb,'GorR') == ' ') % Gap
      |     helpVariable1 = '~=';
      | else % Range
      |     helpVariable1 = '==';
      | end
      | set_param([gcb '/Relational Operator'],'Operator',helpVariable1);
      mask StyleString: popup(Range|Gap  ),edit
      mask Display:
      | port_label('output',1,'A');
      | port_label('input',1,'Sig');
      | port_label('input',2,'Ref');
      | text(0.40,0.53,'+');
      | text(0.415,0.46,'-');
      | text(0.5,0.5,num2str(AbsoluteTolerance));
      | text(0.05,0.5,helpVariable1);
  CC active & no target1 : Subsystem  mask(Range - Gap Absolute Tolerance){GorR=Range, AbsoluteTolerance=0}
      mask prompts: GorR "Use range or gap"; AbsoluteTolerance "Absolute Tolerance"
      mask help: Check that a signal stays inside a range or outside a gap around a reference signal. Specify the range or the gap absolute to the reference signal.
      mask init:
      | if max(get_param(gcb,'GorR') == ' ') % Gap
      |     helpVariable1 = '~=';
      | else % Range
      |     helpVariable1 = '==';
      | end
      | set_param([gcb '/Relational Operator'],'Operator',helpVariable1);
      mask StyleString: popup(Range|Gap  ),edit
      mask Display:
      | port_label('output',1,'A');
      | port_label('input',1,'Sig');
      | port_label('input',2,'Ref');
      | text(0.40,0.53,'+');
      | text(0.415,0.46,'-');
      | text(0.5,0.5,num2str(AbsoluteTolerance));
      | text(0.05,0.5,helpVariable1);
  PS : Subsystem  mask(Feature layer: preconditions synchronization){NoTI=3, NoTDD=0, NoTID=0, TIdel=[0  0  0], TDDdel=[]}
      mask prompts: NoTI "Time-independent features identifiable with or without a delay (TI)"; NoTDD "Triggered features identifiable with determinate delay or without a delay (TDD)"; NoTID "Triggered features identifiable with indeterminate delay (TID)"; TIdel "Time-independent features delays (in time steps). E.g. [0 1 0] for 3 features"; TDDdel "Triggered features delays (in time steps). E.g. [0 0] for 2 features"
      mask help: Use this block for synchronizing the precondition features. For changing the block inputs, use the parameters below. The output must be used for assertions activation.
      mask init:
      | PS_init(gcb);
      mask StyleString: popup(0|1|2|3|4|5|6|7|8|9),popup(0|1|2|3|4|5|6|7|8|9),popup(0|1|2|3|4|5|6|7|8|9),edit,edit
      mask CallbackString:
      | PSTI_callback(gcb);|PSTDD_callback(gcb);|PSTID_callback(gcb);|NoTI = str2double(get_param(gcb,'NoTI'));
      | TIdel = str2num(get_param(gcb,'TIdel'));
      | if NoTI ~= length(TIdel) && NoTI ~= 0
      |     error(['The number of delays entered (' num2str(length(TIdel)) ') does not correspond to the above specified number of time-independent features (' num2str(NoTI) ').']);
      | end|NoTDD = str2double(get_param(gcb,'NoTDD'));
      | TDDdel = str2num(get_param(gcb,'TDDdel'));
      | if NoTDD ~= length(TDDdel) && NoTDD ~= 0
      |     error(['The number of delays entered (' num2str(length(TDDdel)) ') does not correspond to the above specified number of triggered features with constant delay (' num2str(NoTDD) ').']);
      | end
  Scope1 : Scope  NumInputPorts=3
      settings: TimeRange=120  YMin=-0.003370786516853574~-5~-5  YMax=0.3966292134831465~5~5  SaveName=ScopeData5  MaxDataPoints=5000000
  Speed Control active : Subsystem  mask(Range - Gap Absolute Tolerance){GorR=Range, AbsoluteTolerance=0}
      mask prompts: GorR "Use range or gap"; AbsoluteTolerance "Absolute Tolerance"
      mask help: Check that a signal stays inside a range or outside a gap around a reference signal. Specify the range or the gap absolute to the reference signal.
      mask init:
      | if max(get_param(gcb,'GorR') == ' ') % Gap
      |     helpVariable1 = '~=';
      | else % Range
      |     helpVariable1 = '==';
      | end
      | set_param([gcb '/Relational Operator'],'Operator',helpVariable1);
      mask StyleString: popup(Range|Gap  ),edit
      mask Display:
      | port_label('output',1,'A');
      | port_label('input',1,'Sig');
      | port_label('input',2,'Ref');
      | text(0.40,0.53,'+');
      | text(0.415,0.46,'-');
      | text(0.5,0.5,num2str(AbsoluteTolerance));
      | text(0.05,0.5,helpVariable1);
  Step with step size=|1|  and time periods >= 6s detection : Subsystem  mask(Complete step detection){Param=0}
      mask prompts: Param "Mask Parameter 1:"
  true : Constant
  Activate : Outport
  wires:
  PS/1(Precond) -> Activate/1
  InOut Bus/1 -> Bus Selector/1
  Bus Selector/1 -> Step with step size=|1|  and time periods >= 6s detection/1(Step)  "<v_Des>"
  Bus Selector/2 -> CC active & no target/1(Signal)  "<CCMode>"
  Active + no target/1 -> CC active & no target/2(Reference)
  Active/1 -> Speed Control active/2(Reference)
  Bus Selector/3 -> Speed Control active/1(Signal)  "<Selection>"
  Step with step size=|1|  and time periods >= 6s detection/1(Complete step) -> CC active & no target1/1(Signal)
  true/1 -> CC active & no target1/2(Reference)
  CC active & no target1/1(Activate) -> PS/1(A TI1)
  CC active & no target/1(Activate) -> PS/2(A TI2)
  Speed Control active/1(Activate) -> PS/3(A TI3)
